simulink model "decentralized_dead"  (R2023b)
settings: Solver=ode45  StartTime=0.0  StopTime=Tf  RelTol=1e-3
undefined symbols (not defined in the file): A_an2, A_an3, Ac_mrs2, Ac_mrs3, alpha, b, B_an2, B_an3, Bc_mrs2, Bc_mrs3, C2, C3, C_an2, C_an3, C_opt, Cc_mrs2, Cc_mrs3, D_an2, D_an3, Dc_mrs2, Dc_mrs3, p01, p02, p03, p04, phi02, phi03, r_pd1, r_pd2, r_pd3, r_pd4, t1, t2, t3, th, th02, th03, u_max_n1, u_max_n2, u_max_n3, u_max_n4, W_an02, W_an03, xan02, xan03, xc02, xc03, xopt0
settings Model: Creator=lorenzo  LastModifiedBy=lorenzo
settings SolverCC: ZeroCrossControl=DisableAll
settings DebuggingCC: IgnoredZcDiagnostic=none

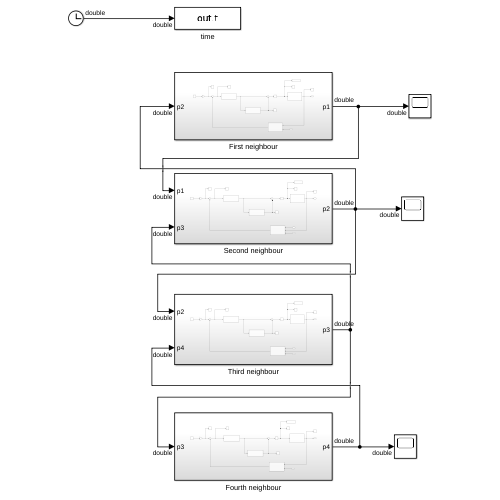
[thumbnail: Simulink's stored preview of the top-level diagram]
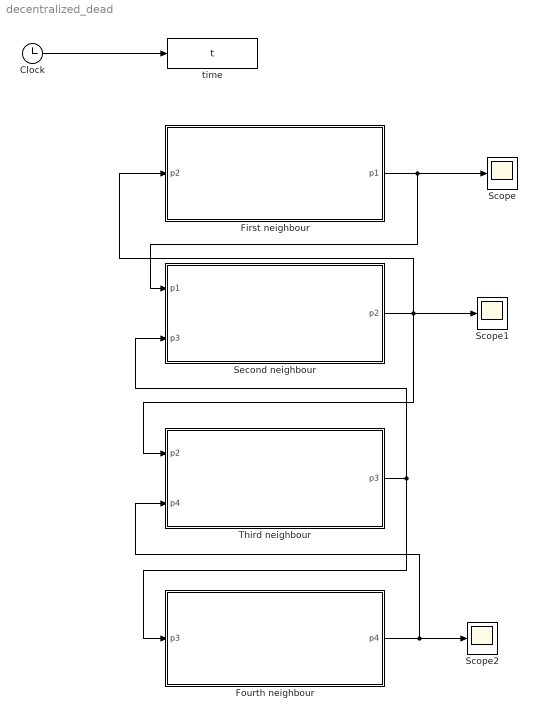
== system decentralized_dead ==
  Clock : Clock
  First neighbour : Subsystem
  Fourth neighbour : Subsystem
  Scope : Scope
  Scope1 : Scope
  Scope2 : Scope
  Second neighbour : Subsystem
  Third neighbour : Subsystem
  time : ToWorkspace  VariableName=t  SampleTime=-1
  wires:
  First neighbour/1(p1) -> Second neighbour/1(p1), Scope/1
  Clock/1 -> time/1
  Second neighbour/1(p2) -> Third neighbour/1(p2), Scope1/1, First neighbour/1(p2)
  Fourth neighbour/1(p4) -> Third neighbour/2(p4), Scope2/1
  Third neighbour/1(p3) -> Fourth neighbour/1(p3), Second neighbour/2(p3)

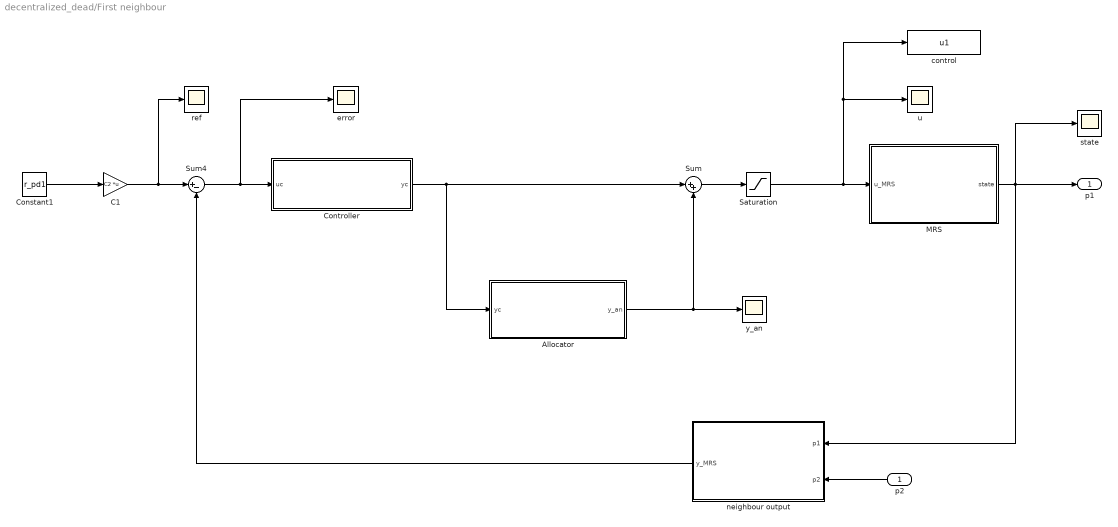
== system decentralized_dead/First neighbour ==
  p2 : Inport
  Allocator : Subsystem
  C1 : Gain  Gain=C2  Multiplication=Matrix(K*u) (u vector)
  Constant1 : Constant  Value=r_pd1  VectorParams1D=off
  Controller : Subsystem
  MRS : Subsystem
  Saturation : Saturate  UpperLimit=u_max_n1  LowerLimit=-u_max_n1
  Sum : Sum  Inputs=|++
  Sum4 : Sum  Inputs=|+-
  control : ToWorkspace  VariableName=u1  SampleTime=-1
  error : Scope
  neighbour output : Subsystem
  ref : Scope
  state : Scope
  u : Scope
  y_an : Scope
  p1 : Outport
  wires:
  Sum4/1 -> error/1, Controller/1(uc)
  MRS/1(state) -> p1/1, neighbour output/1(p1), state/1
  neighbour output/1(y_MRS) -> Sum4/2
  p2/1 -> neighbour output/2(p2)
  Saturation/1 -> MRS/1(u_MRS), control/1, u/1
  Allocator/1(y_an) -> Sum/2, y_an/1
  Controller/1(yc) -> Allocator/1(yc), Sum/1
  Sum/1 -> Saturation/1
  C1/1 -> ref/1, Sum4/1
  Constant1/1 -> C1/1

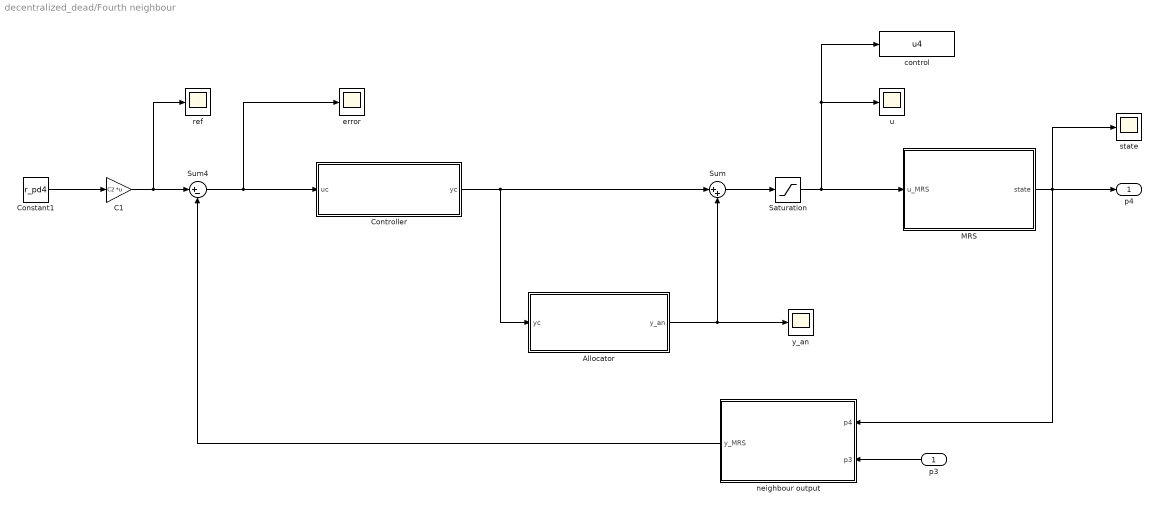
== system decentralized_dead/Fourth neighbour ==
  p3 : Inport
  Allocator : Subsystem
  C1 : Gain  Gain=C2  Multiplication=Matrix(K*u) (u vector)
  Constant1 : Constant  Value=r_pd4  VectorParams1D=off
  Controller : Subsystem
  MRS : Subsystem
  Saturation : Saturate  UpperLimit=u_max_n4  LowerLimit=-u_max_n4
  Sum : Sum  Inputs=|++
  Sum4 : Sum  Inputs=|+-
  control : ToWorkspace  VariableName=u4  SampleTime=-1
  error : Scope
  neighbour output : Subsystem
  ref : Scope
  state : Scope
  u : Scope
  y_an : Scope
  p4 : Outport
  wires:
  Sum4/1 -> error/1, Controller/1(uc)
  MRS/1(state) -> neighbour output/1(p4), state/1, p4/1
  neighbour output/1(y_MRS) -> Sum4/2
  p3/1 -> neighbour output/2(p3)
  Saturation/1 -> control/1, u/1, MRS/1(u_MRS)
  Controller/1(yc) -> Sum/1, Allocator/1(yc)
  Allocator/1(y_an) -> Sum/2, y_an/1
  Sum/1 -> Saturation/1
  Constant1/1 -> C1/1
  C1/1 -> ref/1, Sum4/1

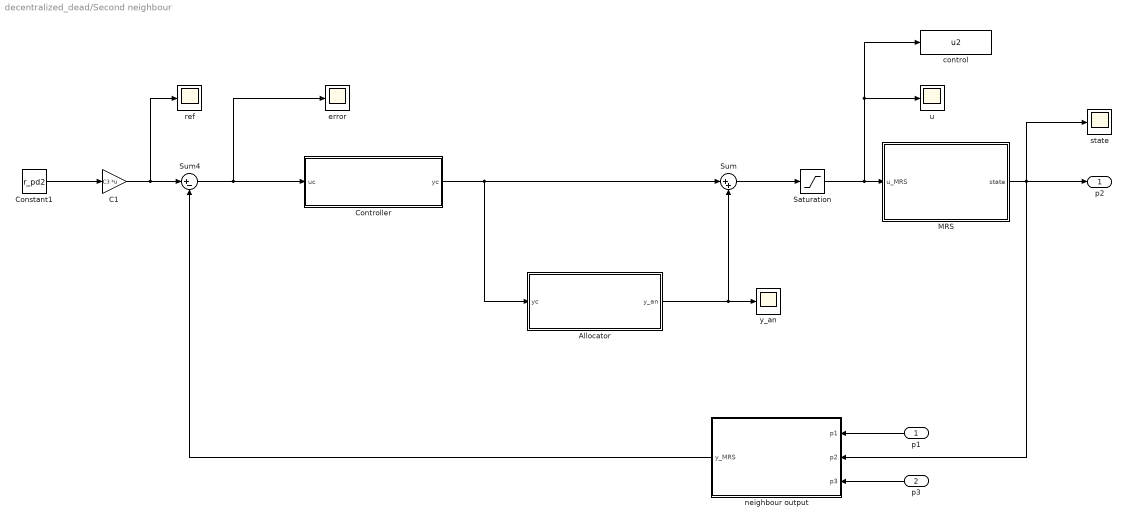
== system decentralized_dead/Second neighbour ==
  p1 : Inport
  p3 : Inport  Port=2
  Allocator : Subsystem
  C1 : Gain  Gain=C3  Multiplication=Matrix(K*u) (u vector)
  Constant1 : Constant  Value=r_pd2  VectorParams1D=off
  Controller : Subsystem
  MRS : Subsystem
  Saturation : Saturate  UpperLimit=u_max_n2  LowerLimit=-u_max_n2
  Sum : Sum  Inputs=|++
  Sum4 : Sum  Inputs=|+-
  control : ToWorkspace  VariableName=u2  SampleTime=-1
  error : Scope
  neighbour output : Subsystem
  ref : Scope
  state : Scope
  u : Scope
  y_an : Scope
  p2 : Outport
  wires:
  Sum4/1 -> error/1, Controller/1(uc)
  MRS/1(state) -> neighbour output/2(p2), state/1, p2/1
  neighbour output/1(y_MRS) -> Sum4/2
  p3/1 -> neighbour output/3(p3)
  p1/1 -> neighbour output/1(p1)
  Saturation/1 -> MRS/1(u_MRS), control/1, u/1
  Sum/1 -> Saturation/1
  Controller/1(yc) -> Allocator/1(yc), Sum/1
  Allocator/1(y_an) -> Sum/2, y_an/1
  C1/1 -> ref/1, Sum4/1
  Constant1/1 -> C1/1

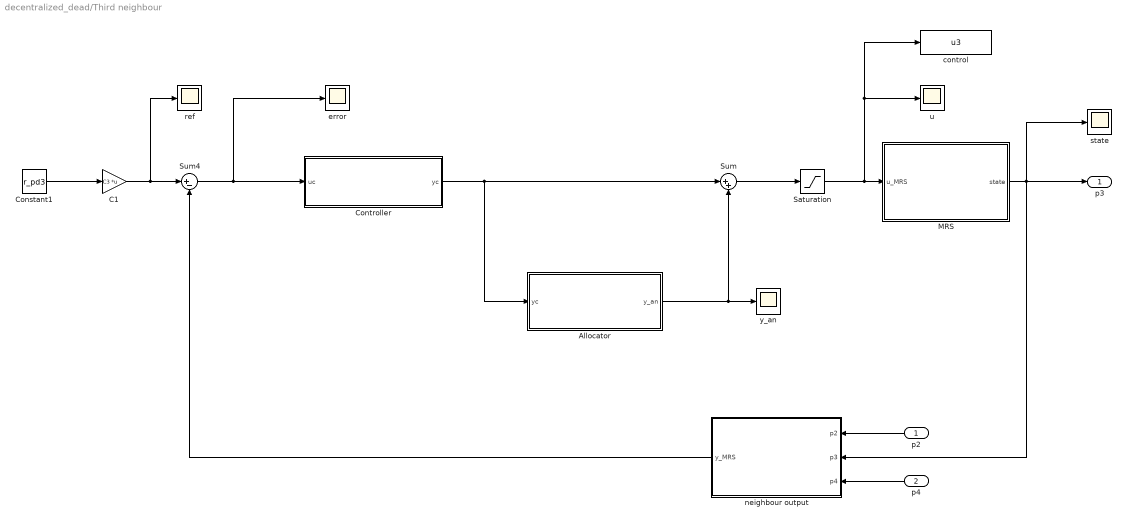
== system decentralized_dead/Third neighbour ==
  p2 : Inport
  p4 : Inport  Port=2
  Allocator : Subsystem
  C1 : Gain  Gain=C3  Multiplication=Matrix(K*u) (u vector)
  Constant1 : Constant  Value=r_pd3  VectorParams1D=off
  Controller : Subsystem
  MRS : Subsystem
  Saturation : Saturate  UpperLimit=u_max_n3  LowerLimit=-u_max_n3
  Sum : Sum  Inputs=|++
  Sum4 : Sum  Inputs=|+-
  control : ToWorkspace  VariableName=u3  SampleTime=-1
  error : Scope
  neighbour output : Subsystem
  ref : Scope
  state : Scope
  u : Scope
  y_an : Scope
  p3 : Outport
  wires:
  Sum4/1 -> error/1, Controller/1(uc)
  MRS/1(state) -> neighbour output/2(p3), state/1, p3/1
  neighbour output/1(y_MRS) -> Sum4/2
  p4/1 -> neighbour output/3(p4)
  p2/1 -> neighbour output/1(p2)
  Saturation/1 -> MRS/1(u_MRS), control/1, u/1
  Sum/1 -> Saturation/1
  Controller/1(yc) -> Allocator/1(yc), Sum/1
  Allocator/1(y_an) -> Sum/2, y_an/1
  C1/1 -> ref/1, Sum4/1
  Constant1/1 -> C1/1

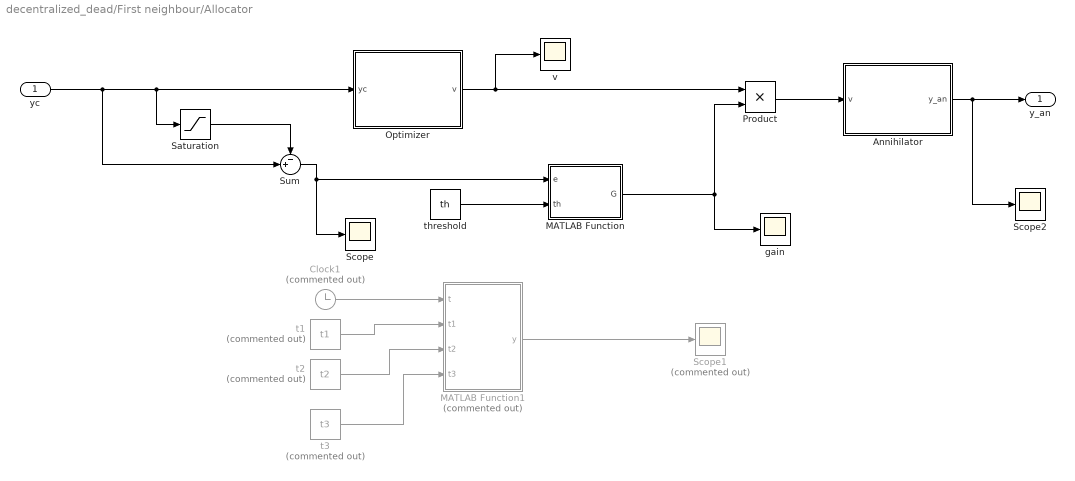
== system decentralized_dead/First neighbour/Allocator ==
  yc : Inport
  Annihilator : Subsystem
  Clock1 : Clock  Commented=on
  MATLAB Function : MATLAB Function  TreatAsAtomicUnit=on
  MATLAB Function1 : MATLAB Function  Commented=on  TreatAsAtomicUnit=on
  Optimizer : Subsystem
  Product : Product
  Saturation : Saturate  UpperLimit=u_max_n1  LowerLimit=-u_max_n1
  Scope : Scope
  Scope1 : Scope  Commented=on
  Scope2 : Scope
  Sum : Sum  Inputs=-+|
  gain : Scope
  t1 : Constant  Commented=on  Value=t1  VectorParams1D=off
  t2 : Constant  Commented=on  Value=t2  VectorParams1D=off
  t3 : Constant  Commented=on  Value=t3  VectorParams1D=off
  threshold : Constant  Value=th
  v : Scope
  y_an : Outport
  wires:
  threshold/1 -> MATLAB Function/2(th)
  yc/1 -> Sum/2, Optimizer/1(yc), Saturation/1
  Product/1 -> Annihilator/1(v)
  Annihilator/1(y_an) -> Scope2/1, y_an/1
  MATLAB Function/1(G) -> Product/2, gain/1
  Optimizer/1(v) -> v/1, Product/1
  Clock1/1 -> MATLAB Function1/1(t)
  t1/1 -> MATLAB Function1/2(t1)
  t2/1 -> MATLAB Function1/3(t2)
  t3/1 -> MATLAB Function1/4(t3)
  MATLAB Function1/1(y) -> Scope1/1
  Saturation/1 -> Sum/1
  Sum/1 -> MATLAB Function/1(e), Scope/1

== system decentralized_dead/First neighbour/Controller ==
  uc : Inport
  Controller formation : Subsystem
  yc : Outport
  wires:
  uc/1 -> Controller formation/1(uc)
  Controller formation/1(u) -> yc/1

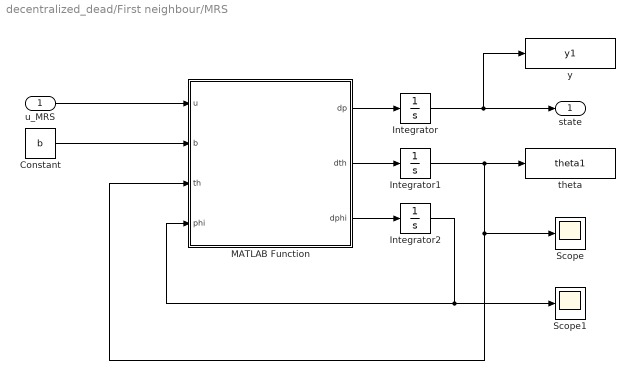
== system decentralized_dead/First neighbour/MRS ==
  u_MRS : Inport
  Constant : Constant  Value=b
  Integrator : Integrator  InitialCondition=p01
  Integrator1 : Integrator  InitialCondition=th02
  Integrator2 : Integrator  InitialCondition=phi02
  MATLAB Function : MATLAB Function  TreatAsAtomicUnit=on
  Scope : Scope
  Scope1 : Scope
  theta : ToWorkspace  VariableName=theta1  SampleTime=-1
  y : ToWorkspace  VariableName=y1  SampleTime=-1
  state : Outport
  wires:
  u_MRS/1 -> MATLAB Function/1(u)
  Constant/1 -> MATLAB Function/2(b)
  MATLAB Function/2(dth) -> Integrator1/1
  MATLAB Function/1(dp) -> Integrator/1
  Integrator1/1 -> MATLAB Function/3(th), Scope/1, theta/1
  MATLAB Function/3(dphi) -> Integrator2/1
  Integrator2/1 -> Scope1/1, MATLAB Function/4(phi)
  Integrator/1 -> y/1, state/1

== system decentralized_dead/First neighbour/neighbour output ==
  p1 : Inport
  p2 : Inport  Port=2
  C : Gain  Gain=C2  Multiplication=Matrix(K*u) (u vector)
  MATLAB Function : MATLAB Function  TreatAsAtomicUnit=on
  y_MRS : Outport
  wires:
  C/1 -> y_MRS/1
  p1/1 -> MATLAB Function/1(y1)
  p2/1 -> MATLAB Function/2(y2)
  MATLAB Function/1(yn) -> C/1

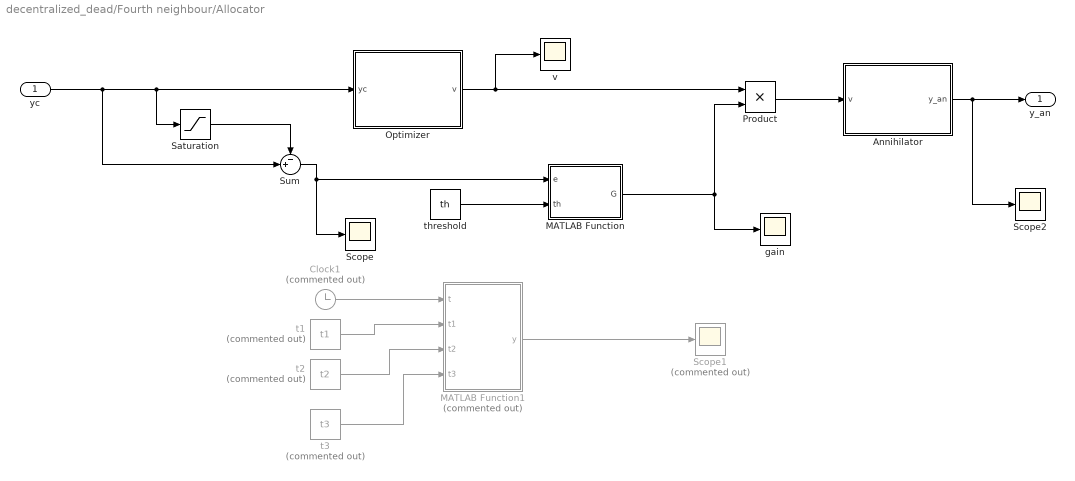
== system decentralized_dead/Fourth neighbour/Allocator ==
  yc : Inport
  Annihilator : Subsystem
  Clock1 : Clock  Commented=on
  MATLAB Function : MATLAB Function  TreatAsAtomicUnit=on
  MATLAB Function1 : MATLAB Function  Commented=on  TreatAsAtomicUnit=on
  Optimizer : Subsystem
  Product : Product
  Saturation : Saturate  UpperLimit=u_max_n4  LowerLimit=-u_max_n4
  Scope : Scope
  Scope1 : Scope  Commented=on
  Scope2 : Scope
  Sum : Sum  Inputs=-+|
  gain : Scope
  t1 : Constant  Commented=on  Value=t1  VectorParams1D=off
  t2 : Constant  Commented=on  Value=t2  VectorParams1D=off
  t3 : Constant  Commented=on  Value=t3  VectorParams1D=off
  threshold : Constant  Value=th
  v : Scope
  y_an : Outport
  wires:
  threshold/1 -> MATLAB Function/2(th)
  yc/1 -> Sum/2, Optimizer/1(yc), Saturation/1
  Product/1 -> Annihilator/1(v)
  Annihilator/1(y_an) -> Scope2/1, y_an/1
  MATLAB Function/1(G) -> Product/2, gain/1
  Optimizer/1(v) -> v/1, Product/1
  Clock1/1 -> MATLAB Function1/1(t)
  t1/1 -> MATLAB Function1/2(t1)
  t2/1 -> MATLAB Function1/3(t2)
  t3/1 -> MATLAB Function1/4(t3)
  MATLAB Function1/1(y) -> Scope1/1
  Saturation/1 -> Sum/1
  Sum/1 -> MATLAB Function/1(e), Scope/1

== system decentralized_dead/Fourth neighbour/Controller ==
  uc : Inport
  Controller formation : Subsystem
  yc : Outport
  wires:
  uc/1 -> Controller formation/1(uc)
  Controller formation/1(u) -> yc/1

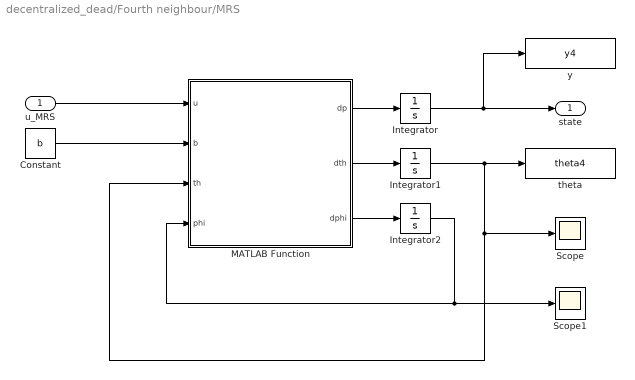
== system decentralized_dead/Fourth neighbour/MRS ==
  u_MRS : Inport
  Constant : Constant  Value=b
  Integrator : Integrator  InitialCondition=p04
  Integrator1 : Integrator  InitialCondition=th03
  Integrator2 : Integrator  InitialCondition=phi03
  MATLAB Function : MATLAB Function  TreatAsAtomicUnit=on
  Scope : Scope
  Scope1 : Scope
  theta : ToWorkspace  VariableName=theta4  SampleTime=-1
  y : ToWorkspace  VariableName=y4  SampleTime=-1
  state : Outport
  wires:
  u_MRS/1 -> MATLAB Function/1(u)
  Constant/1 -> MATLAB Function/2(b)
  MATLAB Function/2(dth) -> Integrator1/1
  MATLAB Function/1(dp) -> Integrator/1
  Integrator1/1 -> MATLAB Function/3(th), Scope/1, theta/1
  MATLAB Function/3(dphi) -> Integrator2/1
  Integrator2/1 -> Scope1/1, MATLAB Function/4(phi)
  Integrator/1 -> y/1, state/1

== system decentralized_dead/Fourth neighbour/neighbour output ==
  p4 : Inport
  p3 : Inport  Port=2
  C : Gain  Gain=C2  Multiplication=Matrix(K*u) (u vector)
  MATLAB Function : MATLAB Function  TreatAsAtomicUnit=on
  y_MRS : Outport
  wires:
  C/1 -> y_MRS/1
  MATLAB Function/1(yn) -> C/1
  p3/1 -> MATLAB Function/1(y1)
  p4/1 -> MATLAB Function/2(y2)

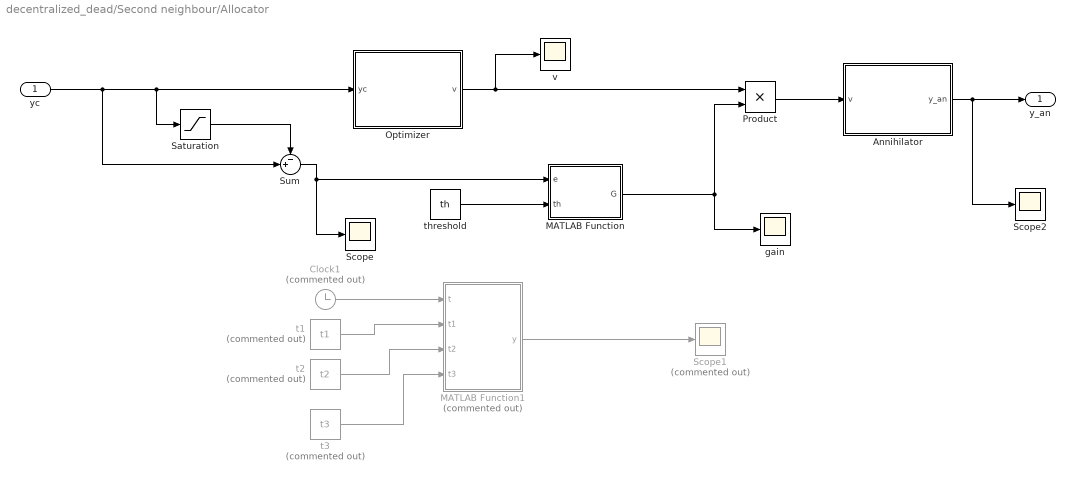
== system decentralized_dead/Second neighbour/Allocator ==
  yc : Inport
  Annihilator : Subsystem
  Clock1 : Clock  Commented=on
  MATLAB Function : MATLAB Function  TreatAsAtomicUnit=on
  MATLAB Function1 : MATLAB Function  Commented=on  TreatAsAtomicUnit=on
  Optimizer : Subsystem
  Product : Product
  Saturation : Saturate  UpperLimit=u_max_n2  LowerLimit=-u_max_n2
  Scope : Scope
  Scope1 : Scope  Commented=on
  Scope2 : Scope
  Sum : Sum  Inputs=-+|
  gain : Scope
  t1 : Constant  Commented=on  Value=t1  VectorParams1D=off
  t2 : Constant  Commented=on  Value=t2  VectorParams1D=off
  t3 : Constant  Commented=on  Value=t3  VectorParams1D=off
  threshold : Constant  Value=th
  v : Scope
  y_an : Outport
  wires:
  threshold/1 -> MATLAB Function/2(th)
  yc/1 -> Sum/2, Optimizer/1(yc), Saturation/1
  Product/1 -> Annihilator/1(v)
  Annihilator/1(y_an) -> Scope2/1, y_an/1
  MATLAB Function/1(G) -> Product/2, gain/1
  Optimizer/1(v) -> v/1, Product/1
  Clock1/1 -> MATLAB Function1/1(t)
  t1/1 -> MATLAB Function1/2(t1)
  t2/1 -> MATLAB Function1/3(t2)
  t3/1 -> MATLAB Function1/4(t3)
  MATLAB Function1/1(y) -> Scope1/1
  Saturation/1 -> Sum/1
  Sum/1 -> MATLAB Function/1(e), Scope/1

== system decentralized_dead/Second neighbour/Controller ==
  uc : Inport
  Controller formation : Subsystem
  yc : Outport
  wires:
  uc/1 -> Controller formation/1(uc)
  Controller formation/1(u) -> yc/1

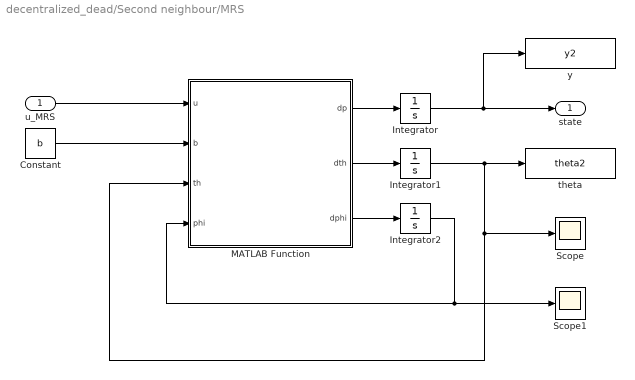
== system decentralized_dead/Second neighbour/MRS ==
  u_MRS : Inport
  Constant : Constant  Value=b
  Integrator : Integrator  InitialCondition=p02
  Integrator1 : Integrator  InitialCondition=th02
  Integrator2 : Integrator  InitialCondition=phi02
  MATLAB Function : MATLAB Function  TreatAsAtomicUnit=on
  Scope : Scope
  Scope1 : Scope
  theta : ToWorkspace  VariableName=theta2  SampleTime=-1
  y : ToWorkspace  VariableName=y2  SampleTime=-1
  state : Outport
  wires:
  u_MRS/1 -> MATLAB Function/1(u)
  Constant/1 -> MATLAB Function/2(b)
  MATLAB Function/2(dth) -> Integrator1/1
  MATLAB Function/1(dp) -> Integrator/1
  Integrator1/1 -> MATLAB Function/3(th), Scope/1, theta/1
  MATLAB Function/3(dphi) -> Integrator2/1
  Integrator2/1 -> Scope1/1, MATLAB Function/4(phi)
  Integrator/1 -> y/1, state/1

== system decentralized_dead/Second neighbour/neighbour output ==
  p1 : Inport
  p2 : Inport  Port=2
  p3 : Inport  Port=3
  C : Gain  Gain=C3  Multiplication=Matrix(K*u) (u vector)
  MATLAB Function : MATLAB Function  TreatAsAtomicUnit=on
  y_MRS : Outport
  wires:
  C/1 -> y_MRS/1
  MATLAB Function/1(yn) -> C/1
  p3/1 -> MATLAB Function/3(y3)
  p2/1 -> MATLAB Function/2(y2)
  p1/1 -> MATLAB Function/1(y1)

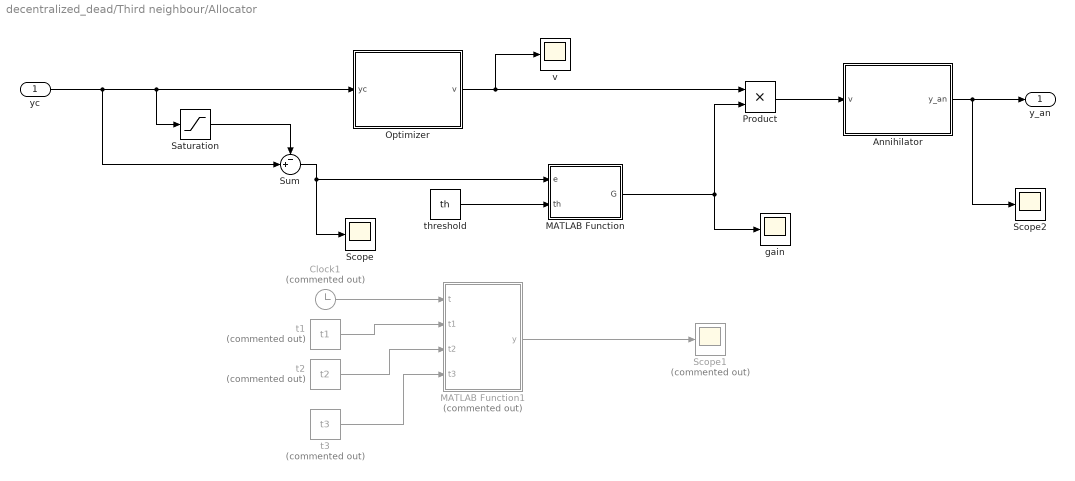
== system decentralized_dead/Third neighbour/Allocator ==
  yc : Inport
  Annihilator : Subsystem
  Clock1 : Clock  Commented=on
  MATLAB Function : MATLAB Function  TreatAsAtomicUnit=on
  MATLAB Function1 : MATLAB Function  Commented=on  TreatAsAtomicUnit=on
  Optimizer : Subsystem
  Product : Product
  Saturation : Saturate  UpperLimit=u_max_n3  LowerLimit=-u_max_n3
  Scope : Scope
  Scope1 : Scope  Commented=on
  Scope2 : Scope
  Sum : Sum  Inputs=-+|
  gain : Scope
  t1 : Constant  Commented=on  Value=t1  VectorParams1D=off
  t2 : Constant  Commented=on  Value=t2  VectorParams1D=off
  t3 : Constant  Commented=on  Value=t3  VectorParams1D=off
  threshold : Constant  Value=th
  v : Scope
  y_an : Outport
  wires:
  threshold/1 -> MATLAB Function/2(th)
  yc/1 -> Sum/2, Optimizer/1(yc), Saturation/1
  Product/1 -> Annihilator/1(v)
  Annihilator/1(y_an) -> Scope2/1, y_an/1
  MATLAB Function/1(G) -> Product/2, gain/1
  Optimizer/1(v) -> v/1, Product/1
  Clock1/1 -> MATLAB Function1/1(t)
  t1/1 -> MATLAB Function1/2(t1)
  t2/1 -> MATLAB Function1/3(t2)
  t3/1 -> MATLAB Function1/4(t3)
  MATLAB Function1/1(y) -> Scope1/1
  Saturation/1 -> Sum/1
  Sum/1 -> MATLAB Function/1(e), Scope/1

== system decentralized_dead/Third neighbour/Controller ==
  uc : Inport
  Controller formation : Subsystem
  yc : Outport
  wires:
  uc/1 -> Controller formation/1(uc)
  Controller formation/1(u) -> yc/1

== system decentralized_dead/Third neighbour/MRS ==
  u_MRS : Inport
  Constant : Constant  Value=b
  Integrator : Integrator  InitialCondition=p03
  Integrator1 : Integrator  InitialCondition=th03
  Integrator2 : Integrator  InitialCondition=phi03
  MATLAB Function : MATLAB Function  TreatAsAtomicUnit=on
  Scope : Scope
  Scope1 : Scope
  theta : ToWorkspace  VariableName=theta3  SampleTime=-1
  y : ToWorkspace  VariableName=y3  SampleTime=-1
  state : Outport
  wires:
  u_MRS/1 -> MATLAB Function/1(u)
  Constant/1 -> MATLAB Function/2(b)
  MATLAB Function/2(dth) -> Integrator1/1
  MATLAB Function/1(dp) -> Integrator/1
  Integrator1/1 -> MATLAB Function/3(th), Scope/1, theta/1
  MATLAB Function/3(dphi) -> Integrator2/1
  Integrator2/1 -> Scope1/1, MATLAB Function/4(phi)
  Integrator/1 -> y/1, state/1

== system decentralized_dead/Third neighbour/neighbour output ==
  p2 : Inport
  p3 : Inport  Port=2
  p4 : Inport  Port=3
  C : Gain  Gain=C3  Multiplication=Matrix(K*u) (u vector)
  MATLAB Function : MATLAB Function  TreatAsAtomicUnit=on
  y_MRS : Outport
  wires:
  C/1 -> y_MRS/1
  MATLAB Function/1(yn) -> C/1
  p4/1 -> MATLAB Function/3(y3)
  p3/1 -> MATLAB Function/2(y2)
  p2/1 -> MATLAB Function/1(y1)

== system decentralized_dead/First neighbour/Allocator/Annihilator ==
  v : Inport
  A_an : Gain  Gain=A_an2  Multiplication=Matrix(K*u) (u vector)
  B_an : Gain  Gain=B_an2  Multiplication=Matrix(K*u) (u vector)
  C_an : Gain  Gain=C_an2  Multiplication=Matrix(K*u) (u vector)
  D_an : Gain  Gain=D_an2  Multiplication=Matrix(K*u) (u vector)
  Integrator : Integrator  InitialCondition=xan02
  Sum : Sum  Inputs=|++
  Sum1 : Sum  Inputs=++|
  y_an1 : ToWorkspace  VariableName=yan1  SampleTime=-1
  y_an : Outport
  wires:
  Integrator/1 -> C_an/1, A_an/1
  B_an/1 -> Sum/2
  A_an/1 -> Sum/1
  Sum/1 -> Integrator/1
  C_an/1 -> Sum1/2
  D_an/1 -> Sum1/1
  Sum1/1 -> y_an1/1, y_an/1
  v/1 -> B_an/1, D_an/1

== system decentralized_dead/First neighbour/Allocator/Optimizer ==
  yc : Inport
  C_opt : Gain  Gain=C_opt  Multiplication=Matrix(K*u) (u vector)
  Constant : Constant  Value=alpha
  Integrator : Integrator  InitialCondition=xopt0
  Wan0 : Constant  Value=W_an02  VectorParams1D=off
  dx_opt : MATLAB Function  TreatAsAtomicUnit=on
  u_max : Constant  Value=u_max_n1
  v : Outport
  wires:
  Integrator/1 -> C_opt/1, dx_opt/4(x_opt)
  dx_opt/1(dx_opt) -> Integrator/1
  C_opt/1 -> v/1
  Constant/1 -> dx_opt/1(alpha)
  yc/1 -> dx_opt/2(yc)
  Wan0/1 -> dx_opt/3(Wan0)
  u_max/1 -> dx_opt/5(u_max)

== system decentralized_dead/First neighbour/Controller/Controller formation ==
  uc : Inport
  Ac_mrs : Gain  Gain=Ac_mrs2  Multiplication=Matrix(K*u) (u vector)
  Bc_mrs : Gain  Gain=Bc_mrs2  Multiplication=Matrix(K*u) (u vector)
  Cc_mrs : Gain  Gain=Cc_mrs2  Multiplication=Matrix(K*u) (u vector)
  Dc_mrs : Gain  Gain=Dc_mrs2  Multiplication=Matrix(K*u) (u vector)
  Integrator : Integrator  InitialCondition=xc02
  Sum : Sum  Inputs=|++
  Sum1 : Sum  Inputs=++|
  u : Outport
  wires:
  Bc_mrs/1 -> Sum1/1
  Cc_mrs/1 -> Sum/1
  uc/1 -> Bc_mrs/1, Dc_mrs/1
  Integrator/1 -> Ac_mrs/1, Cc_mrs/1
  Dc_mrs/1 -> Sum/2
  Sum/1 -> u/1
  Ac_mrs/1 -> Sum1/2
  Sum1/1 -> Integrator/1

== system decentralized_dead/Fourth neighbour/Allocator/Annihilator ==
  v : Inport
  A_an : Gain  Gain=A_an2  Multiplication=Matrix(K*u) (u vector)
  B_an : Gain  Gain=B_an2  Multiplication=Matrix(K*u) (u vector)
  C_an : Gain  Gain=C_an2  Multiplication=Matrix(K*u) (u vector)
  D_an : Gain  Gain=D_an2  Multiplication=Matrix(K*u) (u vector)
  Integrator : Integrator  InitialCondition=xan02
  Sum : Sum  Inputs=|++
  Sum1 : Sum  Inputs=++|
  y_an1 : ToWorkspace  VariableName=yan4  SampleTime=-1
  y_an : Outport
  wires:
  Integrator/1 -> C_an/1, A_an/1
  B_an/1 -> Sum/2
  A_an/1 -> Sum/1
  Sum/1 -> Integrator/1
  C_an/1 -> Sum1/2
  D_an/1 -> Sum1/1
  Sum1/1 -> y_an1/1, y_an/1
  v/1 -> B_an/1, D_an/1

== system decentralized_dead/Fourth neighbour/Allocator/Optimizer ==
  yc : Inport
  C_opt : Gain  Gain=C_opt  Multiplication=Matrix(K*u) (u vector)
  Constant : Constant  Value=alpha
  Integrator : Integrator  InitialCondition=xopt0
  Wan0 : Constant  Value=W_an02  VectorParams1D=off
  dx_opt : MATLAB Function  TreatAsAtomicUnit=on
  u_max : Constant  Value=u_max_n4
  v : Outport
  wires:
  Integrator/1 -> C_opt/1, dx_opt/4(x_opt)
  dx_opt/1(dx_opt) -> Integrator/1
  C_opt/1 -> v/1
  Constant/1 -> dx_opt/1(alpha)
  yc/1 -> dx_opt/2(yc)
  Wan0/1 -> dx_opt/3(Wan0)
  u_max/1 -> dx_opt/5(u_max)

== system decentralized_dead/Fourth neighbour/Controller/Controller formation ==
  uc : Inport
  Ac_mrs : Gain  Gain=Ac_mrs2  Multiplication=Matrix(K*u) (u vector)
  Bc_mrs : Gain  Gain=Bc_mrs2  Multiplication=Matrix(K*u) (u vector)
  Cc_mrs : Gain  Gain=Cc_mrs2  Multiplication=Matrix(K*u) (u vector)
  Dc_mrs : Gain  Gain=Dc_mrs2  Multiplication=Matrix(K*u) (u vector)
  Integrator : Integrator  InitialCondition=xc02
  Sum : Sum  Inputs=|++
  Sum1 : Sum  Inputs=++|
  u : Outport
  wires:
  Bc_mrs/1 -> Sum1/1
  Cc_mrs/1 -> Sum/1
  uc/1 -> Bc_mrs/1, Dc_mrs/1
  Integrator/1 -> Ac_mrs/1, Cc_mrs/1
  Dc_mrs/1 -> Sum/2
  Sum/1 -> u/1
  Ac_mrs/1 -> Sum1/2
  Sum1/1 -> Integrator/1

== system decentralized_dead/Second neighbour/Allocator/Annihilator ==
  v : Inport
  A_an : Gain  Gain=A_an3  Multiplication=Matrix(K*u) (u vector)
  B_an : Gain  Gain=B_an3  Multiplication=Matrix(K*u) (u vector)
  C_an : Gain  Gain=C_an3  Multiplication=Matrix(K*u) (u vector)
  D_an : Gain  Gain=D_an3  Multiplication=Matrix(K*u) (u vector)
  Integrator : Integrator  InitialCondition=xan03
  Sum : Sum  Inputs=|++
  Sum1 : Sum  Inputs=++|
  y_an1 : ToWorkspace  VariableName=yan2  SampleTime=-1
  y_an : Outport
  wires:
  Integrator/1 -> C_an/1, A_an/1
  B_an/1 -> Sum/2
  A_an/1 -> Sum/1
  Sum/1 -> Integrator/1
  C_an/1 -> Sum1/2
  D_an/1 -> Sum1/1
  Sum1/1 -> y_an1/1, y_an/1
  v/1 -> B_an/1, D_an/1

== system decentralized_dead/Second neighbour/Allocator/Optimizer ==
  yc : Inport
  C_opt : Gain  Gain=C_opt  Multiplication=Matrix(K*u) (u vector)
  Constant : Constant  Value=alpha
  Integrator : Integrator  InitialCondition=xopt0
  Wan0 : Constant  Value=W_an03  VectorParams1D=off
  dx_opt : MATLAB Function  TreatAsAtomicUnit=on
  u_max : Constant  Value=u_max_n2
  v : Outport
  wires:
  Integrator/1 -> C_opt/1, dx_opt/4(x_opt)
  dx_opt/1(dx_opt) -> Integrator/1
  C_opt/1 -> v/1
  Constant/1 -> dx_opt/1(alpha)
  yc/1 -> dx_opt/2(yc)
  Wan0/1 -> dx_opt/3(Wan0)
  u_max/1 -> dx_opt/5(u_max)

== system decentralized_dead/Second neighbour/Controller/Controller formation ==
  uc : Inport
  Ac_mrs : Gain  Gain=Ac_mrs3  Multiplication=Matrix(K*u) (u vector)
  Bc_mrs : Gain  Gain=Bc_mrs3  Multiplication=Matrix(K*u) (u vector)
  Cc_mrs : Gain  Gain=Cc_mrs3  Multiplication=Matrix(K*u) (u vector)
  Dc_mrs : Gain  Gain=Dc_mrs3  Multiplication=Matrix(K*u) (u vector)
  Integrator : Integrator  InitialCondition=xc03
  Sum : Sum  Inputs=|++
  Sum1 : Sum  Inputs=++|
  u : Outport
  wires:
  Bc_mrs/1 -> Sum1/1
  Cc_mrs/1 -> Sum/1
  uc/1 -> Bc_mrs/1, Dc_mrs/1
  Integrator/1 -> Ac_mrs/1, Cc_mrs/1
  Dc_mrs/1 -> Sum/2
  Sum/1 -> u/1
  Ac_mrs/1 -> Sum1/2
  Sum1/1 -> Integrator/1

== system decentralized_dead/Third neighbour/Allocator/Annihilator ==
  v : Inport
  A_an : Gain  Gain=A_an3  Multiplication=Matrix(K*u) (u vector)
  B_an : Gain  Gain=B_an3  Multiplication=Matrix(K*u) (u vector)
  C_an : Gain  Gain=C_an3  Multiplication=Matrix(K*u) (u vector)
  D_an : Gain  Gain=D_an3  Multiplication=Matrix(K*u) (u vector)
  Integrator : Integrator  InitialCondition=xan03
  Sum : Sum  Inputs=|++
  Sum1 : Sum  Inputs=++|
  y_an1 : ToWorkspace  VariableName=yan3  SampleTime=-1
  y_an : Outport
  wires:
  Integrator/1 -> C_an/1, A_an/1
  B_an/1 -> Sum/2
  A_an/1 -> Sum/1
  Sum/1 -> Integrator/1
  C_an/1 -> Sum1/2
  D_an/1 -> Sum1/1
  Sum1/1 -> y_an1/1, y_an/1
  v/1 -> B_an/1, D_an/1

== system decentralized_dead/Third neighbour/Allocator/Optimizer ==
  yc : Inport
  C_opt : Gain  Gain=C_opt  Multiplication=Matrix(K*u) (u vector)
  Constant : Constant  Value=alpha
  Integrator : Integrator  InitialCondition=xopt0
  Wan0 : Constant  Value=W_an03  VectorParams1D=off
  dx_opt : MATLAB Function  TreatAsAtomicUnit=on
  u_max : Constant  Value=u_max_n3
  v : Outport
  wires:
  Integrator/1 -> C_opt/1, dx_opt/4(x_opt)
  dx_opt/1(dx_opt) -> Integrator/1
  C_opt/1 -> v/1
  Constant/1 -> dx_opt/1(alpha)
  yc/1 -> dx_opt/2(yc)
  Wan0/1 -> dx_opt/3(Wan0)
  u_max/1 -> dx_opt/5(u_max)

== system decentralized_dead/Third neighbour/Controller/Controller formation ==
  uc : Inport
  Ac_mrs : Gain  Gain=Ac_mrs3  Multiplication=Matrix(K*u) (u vector)
  Bc_mrs : Gain  Gain=Bc_mrs3  Multiplication=Matrix(K*u) (u vector)
  Cc_mrs : Gain  Gain=Cc_mrs3  Multiplication=Matrix(K*u) (u vector)
  Dc_mrs : Gain  Gain=Dc_mrs3  Multiplication=Matrix(K*u) (u vector)
  Integrator : Integrator  InitialCondition=xc03
  Sum : Sum  Inputs=|++
  Sum1 : Sum  Inputs=++|
  u : Outport
  wires:
  Bc_mrs/1 -> Sum1/1
  Cc_mrs/1 -> Sum/1
  uc/1 -> Bc_mrs/1, Dc_mrs/1
  Integrator/1 -> Ac_mrs/1, Cc_mrs/1
  Dc_mrs/1 -> Sum/2
  Sum/1 -> u/1
  Ac_mrs/1 -> Sum1/2
  Sum1/1 -> Integrator/1

== matlab function decentralized_dead/Fourth neighbour/MRS/MATLAB Function ==
  data: u input; b input; dp output; th input; dth output; phi input; dphi output
function [dp,dth,dphi] = platoon_MRS(u,b,th,phi)

ui = u(3:4);

th1 = th(1);

phi1 = phi(1);

B = eye(2);

Bth = tan(phi1)*[cos(th1) sin(th1)];

Bphi = 1/b*[-sin(th1) cos(th1)];

dp = B*ui;
dth = Bth*ui;
dphi = Bphi*ui;

== matlab function decentralized_dead/Fourth neighbour/neighbour output/MATLAB Function ==
  data: y1 input; yn output; y2 input
function yn = fcn(y1,y2)

yn = [y1;y2];

== matlab function decentralized_dead/First neighbour/neighbour output/MATLAB Function ==
  data: y1 input; yn output; y2 input
function yn = fcn(y1,y2)

yn = [y1;y2];

== matlab function decentralized_dead/First neighbour/Allocator/MATLAB Function ==
  data: e input; G output; th input
function G = fcn(e,th)
norm(e);
eps = th/2;

G=1;

if ( norm(e) < th-eps )
    G = 0;
end
if ( norm(e) > th )
    G = 1;
end
if ( norm(e) <= th && norm(e) >= th-eps )
    G = -2*(norm(e)-(th-eps))^3+3*(norm(e)-(th-eps))^2;
end

== matlab function decentralized_dead/First neighbour/Allocator/MATLAB Function1 ==
  data: t input; y output; t1 input; t2 input; t3 input
function y = reset_sig(t,t1,t2,t3)

y = 1;

if ( t1 < t && t <= t2 )
    y = 0;
elseif ( t2 < t && t <= t3 )
    y = 1;
end

== matlab function decentralized_dead/First neighbour/Allocator/Optimizer/dx_opt ==
  data: dx_opt output; alpha input; yc input; Wan0 input; x_opt input; u_max input
function dx_opt = opt_dyn(alpha,yc,Wan0,x_opt,u_max)

u1_max = u_max(1);
u2_max = u_max(2);
u3_max = u_max(3);
u4_max = u_max(4);

ss_u = yc+Wan0*x_opt;

ss_sat = ss_u;

if ( abs(ss_u(1))>=u1_max )
    ss_sat(1) = sign(ss_u(1))*u1_max;
end
if ( abs(ss_u(2))>=u2_max )
    ss_sat(2) = sign(ss_u(2))*u2_max;
end
if ( abs(ss_u(3))>=u3_max )
    ss_sat(3) = sign(ss_u(3))*u3_max;
end
if ( abs(ss_u(4))>=u4_max )
    ss_sat(4) = sign(ss_u(4))*u4_max;
end

par_der = diag([dsat(ss_u(1),u1_max,0.01),dsat(ss_u(2),u2_max,0.01),dsat(ss_u(3),u3_max,0.01),dsat(ss_u(4),u4_max,0.01)]); 

grad = (yc+Wan0*x_opt-ss_sat)'*(Wan0-par_der*Wan0);

dx_opt = -alpha*grad;

== matlab function decentralized_dead/Fourth neighbour/Allocator/MATLAB Function ==
  data: e input; G output; th input
function G = fcn(e,th)
norm(e);
eps = th/2;

G=1;

if ( norm(e) < th-eps )
    G = 0;
end
if ( norm(e) > th )
    G = 1;
end
if ( norm(e) <= th && norm(e) >= th-eps )
    G = -2*(norm(e)-(th-eps))^3+3*(norm(e)-(th-eps))^2;
end

== matlab function decentralized_dead/Fourth neighbour/Allocator/MATLAB Function1 ==
  data: t input; y output; t1 input; t2 input; t3 input
function y = reset_sig(t,t1,t2,t3)

y = 1;

if ( t1 < t && t <= t2 )
    y = 0;
elseif ( t2 < t && t <= t3 )
    y = 1;
end

== matlab function decentralized_dead/Fourth neighbour/Allocator/Optimizer/dx_opt ==
  data: dx_opt output; alpha input; yc input; Wan0 input; x_opt input; u_max input
function dx_opt = opt_dyn(alpha,yc,Wan0,x_opt,u_max)

u1_max = u_max(1);
u2_max = u_max(2);
u3_max = u_max(3);
u4_max = u_max(4);

ss_u = yc+Wan0*x_opt;

ss_sat = ss_u;

if ( abs(ss_u(1))>=u1_max )
    ss_sat(1) = sign(ss_u(1))*u1_max;
end
if ( abs(ss_u(2))>=u2_max )
    ss_sat(2) = sign(ss_u(2))*u2_max;
end
if ( abs(ss_u(3))>=u3_max )
    ss_sat(3) = sign(ss_u(3))*u3_max;
end
if ( abs(ss_u(4))>=u4_max )
    ss_sat(4) = sign(ss_u(4))*u4_max;
end

par_der = diag([dsat(ss_u(1),u1_max,0.01),dsat(ss_u(2),u2_max,0.01),dsat(ss_u(3),u3_max,0.01),dsat(ss_u(4),u4_max,0.01)]); 

grad = (yc+Wan0*x_opt-ss_sat)'*(Wan0-par_der*Wan0);

dx_opt = -alpha*grad;

== matlab function decentralized_dead/Second neighbour/Allocator/MATLAB Function ==
  data: e input; G output; th input
function G = fcn(e,th)
norm(e);
eps = th/2;

G=1;

if ( norm(e) < th-eps )
    G = 0;
end
if ( norm(e) > th )
    G = 1;
end
if ( norm(e) <= th && norm(e) >= th-eps )
    G = -2*(norm(e)-(th-eps))^3+3*(norm(e)-(th-eps))^2;
end

== matlab function decentralized_dead/Third neighbour/Allocator/MATLAB Function ==
  data: e input; G output; th input
function G = fcn(e,th)
norm(e);
eps = th/2;

G=1;

if ( norm(e) < th-eps )
    G = 0;
end
if ( norm(e) > th )
    G = 1;
end
if ( norm(e) <= th && norm(e) >= th-eps )
    G = -2*(norm(e)-(th-eps))^3+3*(norm(e)-(th-eps))^2;
end

== matlab function decentralized_dead/Second neighbour/Allocator/MATLAB Function1 ==
  data: t input; y output; t1 input; t2 input; t3 input
function y = reset_sig(t,t1,t2,t3)

y = 1;

if ( t1 < t && t <= t2 )
    y = 0;
elseif ( t2 < t && t <= t3 )
    y = 1;
end

== matlab function decentralized_dead/Second neighbour/Allocator/Optimizer/dx_opt ==
  data: dx_opt output; alpha input; yc input; Wan0 input; x_opt input; u_max input
function dx_opt = opt_dyn(alpha,yc,Wan0,x_opt,u_max)

u1_max = u_max(1);
u2_max = u_max(2);
u3_max = u_max(3);
u4_max = u_max(4);
u5_max = u_max(5);
u6_max = u_max(6);

ss_u = yc+Wan0*x_opt;

ss_sat = ss_u;

if ( abs(ss_u(1))>=u1_max )
    ss_sat(1) = sign(ss_u(1))*u1_max;
end
if ( abs(ss_u(2))>=u2_max )
    ss_sat(2) = sign(ss_u(2))*u2_max;
end
if ( abs(ss_u(3))>=u3_max )
    ss_sat(3) = sign(ss_u(3))*u3_max;
end
if ( abs(ss_u(4))>=u4_max )
    ss_sat(4) = sign(ss_u(4))*u4_max;
end
if ( abs(ss_u(5))>=u5_max )
    ss_sat(5) = sign(ss_u(5))*u5_max;
end
if ( abs(ss_u(6))>=u6_max )
    ss_sat(6) = sign(ss_u(6))*u6_max;
end

par_der = diag([dsat(ss_u(1),u1_max,0.01),dsat(ss_u(2),u2_max,0.01),dsat(ss_u(3),u3_max,0.01),dsat(ss_u(4),u4_max,0.01),dsat(ss_u(5),u5_max,0.01),dsat(ss_u(6),u6_max,0.01)]); 

grad = (yc+Wan0*x_opt-ss_sat)'*(Wan0-par_der*Wan0);

dx_opt = -alpha*grad;

== matlab function decentralized_dead/First neighbour/MRS/MATLAB Function ==
  data: u input; b input; dp output; th input; dth output; phi input; dphi output
function [dp,dth,dphi] = platoon_MRS(u,b,th,phi)

ui = u(1:2);

th1 = th(1);

phi1 = phi(1);

B = eye(2);

Bth = tan(phi1)*[cos(th1) sin(th1)];

Bphi = 1/b*[-sin(th1) cos(th1)];

dp = B*ui;
dth = Bth*ui;
dphi = Bphi*ui;

== matlab function decentralized_dead/Third neighbour/Allocator/MATLAB Function1 ==
  data: t input; y output; t1 input; t2 input; t3 input
function y = reset_sig(t,t1,t2,t3)

y = 1;

if ( t1 < t && t <= t2 )
    y = 0;
elseif ( t2 < t && t <= t3 )
    y = 1;
end

== matlab function decentralized_dead/Third neighbour/Allocator/Optimizer/dx_opt ==
  data: dx_opt output; alpha input; yc input; Wan0 input; x_opt input; u_max input
function dx_opt = opt_dyn(alpha,yc,Wan0,x_opt,u_max)

u1_max = u_max(1);
u2_max = u_max(2);
u3_max = u_max(3);
u4_max = u_max(4);
u5_max = u_max(5);
u6_max = u_max(6);

ss_u = yc+Wan0*x_opt;

ss_sat = ss_u;

if ( abs(ss_u(1))>=u1_max )
    ss_sat(1) = sign(ss_u(1))*u1_max;
end
if ( abs(ss_u(2))>=u2_max )
    ss_sat(2) = sign(ss_u(2))*u2_max;
end
if ( abs(ss_u(3))>=u3_max )
    ss_sat(3) = sign(ss_u(3))*u3_max;
end
if ( abs(ss_u(4))>=u4_max )
    ss_sat(4) = sign(ss_u(4))*u4_max;
end
if ( abs(ss_u(5))>=u5_max )
    ss_sat(5) = sign(ss_u(5))*u5_max;
end
if ( abs(ss_u(6))>=u6_max )
    ss_sat(6) = sign(ss_u(6))*u6_max;
end

par_der = diag([dsat(ss_u(1),u1_max,0.01),dsat(ss_u(2),u2_max,0.01),dsat(ss_u(3),u3_max,0.01),dsat(ss_u(4),u4_max,0.01),dsat(ss_u(5),u5_max,0.01),dsat(ss_u(6),u6_max,0.01)]); 

grad = (yc+Wan0*x_opt-ss_sat)'*(Wan0-par_der*Wan0);

dx_opt = -alpha*grad;

== matlab function decentralized_dead/Third neighbour/MRS/MATLAB Function ==
  data: u input; b input; dp output; th input; dth output; phi input; dphi output
function [dp,dth,dphi] = platoon_MRS(u,b,th,phi)

ui = u(3:4);

th1 = th(1);

phi1 = phi(1);

B = eye(2);

Bth = tan(phi1)*[cos(th1) sin(th1)];

Bphi = 1/b*[-sin(th1) cos(th1)];

dp = B*ui;
dth = Bth*ui;
dphi = Bphi*ui;

== matlab function decentralized_dead/Third neighbour/neighbour output/MATLAB Function ==
  data: y1 input; yn output; y2 input; y3 input
function yn = fcn(y1,y2,y3)

yn = [y1;y2;y3];

== matlab function decentralized_dead/Second neighbour/MRS/MATLAB Function ==
  data: u input; b input; dp output; th input; dth output; phi input; dphi output
function [dp,dth,dphi] = platoon_MRS(u,b,th,phi)

ui = u(3:4);

th1 = th(1);

phi1 = phi(1);

B = eye(2);

Bth = tan(phi1)*[cos(th1) sin(th1)];

Bphi = 1/b*[-sin(th1) cos(th1)];

dp = B*ui;
dth = Bth*ui;
dphi = Bphi*ui;

== matlab function decentralized_dead/Second neighbour/neighbour output/MATLAB Function ==
  data: y1 input; yn output; y2 input; y3 input
function yn = fcn(y1,y2,y3)

yn = [y1;y2;y3];
